simulink model "simscape_actuation_22_idealtorque"  (R2021a)
settings: Solver=VariableStepAuto  StartTime=0.001  StopTime=10  FixedStep=0.01  MaxStep=0.0001  RelTol=1e-4  AbsTol=1e-4
values from neighbouring files (symbols this model uses):
  As = 0.00025    [variables_5.mat]
  ext = 48232.2966308    [variables_5.mat]
  n = 0.912908754682    [variables_5.mat]
  ri = 0.00045    [variables_5.mat]
  ro = 0.0015    [variables_5.mat]
  Y = 7920.45919172    [variables_5.mat]
  yieldstress = 40000000    [variables_5.mat]
undefined symbols (not defined in the file or in its folder): Fac
libraries: fl_lib x18, sh_lib x11, nesl_utility x10, sdl_lib x2, pid_lib x1
settings Model: Creator=carme  LastModifiedBy=carme
settings SolverCC: AutoScaleAbsTol=off  AlgebraicLoopSolver=LineSearch
settings DebuggingCC: SymbolicDimsDataTypeCodeGenerationDiagnostic=none  SFMachineParentedDataDiag=warning
settings SFSimCC: CustomCodeUndefinedFunction=UseInterfaceOnly
settings SimscapeCC: SimscapeLogType=all  SimscapeLogSimulationStatistics=on  SimscapeLogDataHistory=10000

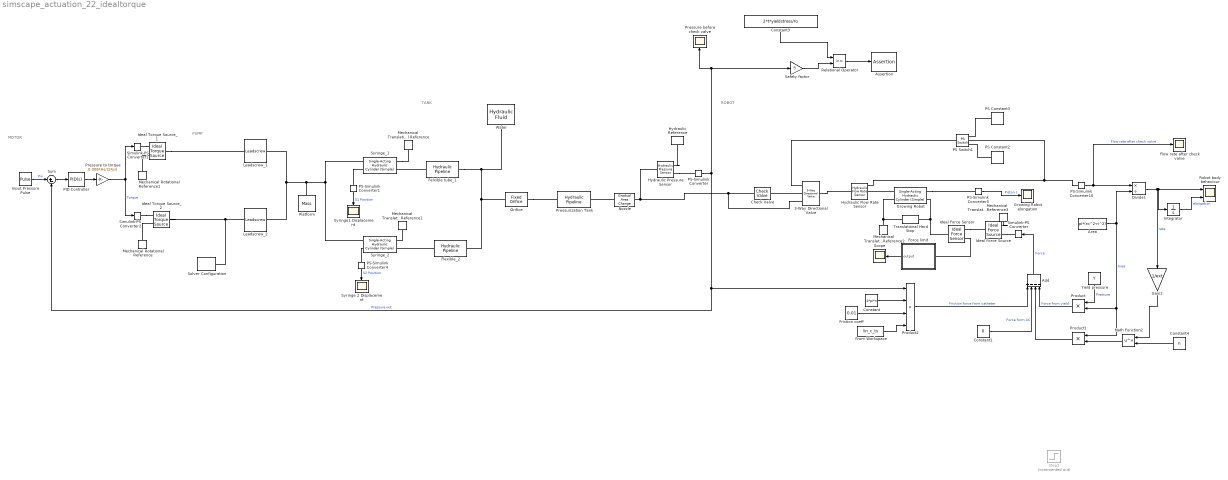
== system simscape_actuation_22_idealtorque ==
  note: MOTOR
  note: PUMP
  note: TANK
  note: ROBOT
  3-Way Directional Valve : sh_lib/Valves/Directional Valves/3-Way Directional Valve  area_spec=sh.valves.directional_valves.enum.area_spec.identical  x_0_P=0 m  x_0_T=0 m  mdl_type_identical=sh.valves.directional_valves.enum.mdl_type.linear  mdl_type_different=sh.valves.directional_valves.enum.mdl_type.linear  opening_max=0.005 m  area_max=0.5e-4 m^2  opening_max_P_A=0.005 m  area_max_P_A=0.5e-4 m^2  opening_max_A_T=0.005 m  area_max_A_T=0.5e-4 m^2  opening_area_tab=[-.002, 0, .002, .005, .015] m  area_tab=[1e-09, 2.0352e-07, 4.0736e-05, .00011438, .00034356] m^2  opening_flow_rate_tab=[-.002, 0, .002, .005, .015] m  pressure_tab=[-10000000, -5000000, -2000000, 2000000, 5000000, 10000000] Pa  flow_rate_tab=[-1e-07, -7.0711e-08, -4.4721e-08, 4.4721e-08, 7.0711e-08, 1e-07; -2.0352e-05, -1.4391e-05, -9.1017e-06, 9.1017e-06, 1.4391e-05, 2.0352e-05; -.0040736, -.0028805, -.0018218, .0018218, .0028805, .0040736; -.011438, -.0080879, -.0051152, .0051152, .0080879, .011438; -.034356, -.024293, -.015364, .015364, .024293, .034356] m^3/s  opening_area_tab_P_A=[-.002, 0, .002, .005, .015] m  area_tab_P_A=[1e-09, 2.0352e-07, 4.0736e-05, .00011438, .00034356] m^2  opening_flow_rate_tab_P_A=[-.002, 0, .002, .005, .015] m  pressure_tab_P_A=[-10000000, -5000000, -2000000, 2000000, 5000000, 10000000] Pa  flow_rate_tab_P_A=[-1e-07, -7.0711e-08, -4.4721e-08, 4.4721e-08, 7.0711e-08, 1e-07; -2.0352e-05, -1.4391e-05, -9.1017e-06, 9.1017e-06, 1.4391e-05, 2.0352e-05; -.0040736, -.0028805, -.0018218, .0018218, .0028805, .0040736; -.011438, -.0080879, -.0051152, .0051152, .0080879, .011438; -.034356, -.024293, -.015364, .015364, .024293, .034356] m^3/s  opening_area_tab_A_T=[-.002, 0, .002, .005, .015] m  area_tab_A_T=[1e-09, 2.0352e-07, 4.0736e-05, .00011438, .00034356] m^2  opening_flow_rate_tab_A_T=[-.002, 0, .002, .005, .015] m  pressure_tab_A_T=[-10000000, -5000000, -2000000, 2000000, 5000000, 10000000] Pa  flow_rate_tab_A_T=[-1e-07, -7.0711e-08, -4.4721e-08, 4.4721e-08, 7.0711e-08, 1e-07; -2.0352e-05, -1.4391e-05, -9.1017e-06, 9.1017e-06, 1.4391e-05, 2.0352e-05; -.0040736, -.0028805, -.0018218, .0018218, .0028805, .0040736; -.011438, -.0080879, -.0051152, .0051152, .0080879, .011438; -.034356, -.024293, -.015364, .015364, .024293, .034356] m^3/s  interp_method_identical=sh.valves.directional_valves.enum.interp_method.linear  interp_method_different=sh.valves.directional_valves.enum.interp_method.linear  extrap_method_identical=sh.valves.directional_valves.enum.extrap_method.linear  extrap_method_different=sh.valves.directional_valves.enum.extrap_method.linear  A_leak=1e-12 m^2  C_d=0.7  lam_spec=sh.valves.directional_valves.enum.lam_spec.pressure_ratio  B_lam=0.999  Re_cr=12
      settings: SourceProductBaseCode=SH  InternalSimscapePortConfiguration="{\"Bottom\":[],\"Left\":[{\"id\":\"A\",\"label\":\"A\",\"type\":\"foundation.hydraulic.hydraulic\"}],\"Right\":[{\"id\":\"S\",\"label\":\"S\",\"type\":\"input\"},{\"id\":\"P\",\"label\":\"P\",\"type\":\"foundation.hydraulic.hydraulic\"},{\"id\":\"T\",\"label\":\"T\",\"type\":\"foundation.hydraulic.hydraulic\"}],\"Top\":[]}"
  Add : Sum  Inputs=+---
  Area : Constant  Value=pi*(ro^2-ri^2)
  Assertion : Assertion  AssertionFailFcn=Yield failure
  Check Valve : sh_lib/Valves/Directional Valves/Check Valve  area_max=As m^2  pres_crack=Y Pa  pres_max=1.2e10 Pa  C_d=0.7  A_leak=1e-12 m^2  lam_spec=1  B_lam=0.999  Re_cr=12  dynamic=0  tau=0.1 s  area_init=1e-12 m^2
      settings: SourceProductBaseCode=SH  InternalSimscapePortConfiguration="{\"Bottom\":[],\"Left\":[{\"id\":\"A\",\"label\":\"A\",\"type\":\"foundation.hydraulic.hydraulic\"}],\"Right\":[{\"id\":\"B\",\"label\":\"B\",\"type\":\"foundation.hydraulic.hydraulic\"}],\"Top\":[]}"
  Constant : Constant  Value=2*pi*ri
  Constant1 : Constant  Value=0
  Constant3 : Constant  Value=2*t*yieldstress/ro
  Constant4 : Constant  Value=n
  Divide1 : Product  Inputs=*/
  Felxible tube_1 : sh_lib/Pipelines/Hydraulic Pipeline  cs_type=1  d_in=0.004 m  area=1e-4 m^2  D_h=1.12e-2 m  s_factor=64  length=0.3 m  length_ad=1 m  roughness=15e-6 m  Re_lam=2000  Re_turb=4000  wall_type=2  pr_r_coef=2e-12 m/Pa  time_const=0.01 s  k_sh=1.4  initial_pressure=200 Pa
      settings: SourceProductBaseCode=SH  InternalSimscapePortConfiguration="{\"Bottom\":[],\"Left\":[{\"id\":\"A\",\"label\":\"A\",\"type\":\"foundation.hydraulic.hydraulic\"}],\"Right\":[{\"id\":\"B\",\"label\":\"B\",\"type\":\"foundation.hydraulic.hydraulic\"}],\"Top\":[]}"
  Flexible_2 : sh_lib/Pipelines/Hydraulic Pipeline  cs_type=1  d_in=0.004 m  area=1e-4 m^2  D_h=1.12e-2 m  s_factor=64  length=0.3 m  length_ad=1 m  roughness=15e-6 m  Re_lam=2000  Re_turb=4000  wall_type=2  pr_r_coef=2e-12 m/Pa  time_const=0.01 s  k_sh=1.4  initial_pressure=200 Pa
      settings: SourceProductBaseCode=SH  InternalSimscapePortConfiguration="{\"Bottom\":[],\"Left\":[{\"id\":\"A\",\"label\":\"A\",\"type\":\"foundation.hydraulic.hydraulic\"}],\"Right\":[{\"id\":\"B\",\"label\":\"B\",\"type\":\"foundation.hydraulic.hydraulic\"}],\"Top\":[]}"
  Flow rate after check valve : Scope
  Force limit : Subsystem  mask{Flim=2}
      mask prompts: Flim "Force limit"
  Friction coeff : Constant  Value=0.01
  From Workspace : FromWorkspace  VariableName=lin_c_ts
  Gain2 : Gain  Gain=1/ext
  Growing Robot : sh_lib/Hydraulic Cylinders/Single-Acting Hydraulic Cylinder (Simple)  area=pi*(ro^2-ri^2) m^2  stroke=0.08 m  init_pos=0.01 m  penetr_coeff=1e12 s*N/m^2  or=1
      settings: SourceProductBaseCode=SH  InternalSimscapePortConfiguration="{\"Bottom\":[],\"Left\":[{\"id\":\"C\",\"label\":\"C\",\"type\":\"foundation.mechanical.translational.translational\"},{\"id\":\"A\",\"label\":\"A\",\"type\":\"foundation.hydraulic.hydraulic\"}],\"Right\":[{\"id\":\"R\",\"label\":\"R\",\"type\":\"foundation.mechanical.translational.translational\"},{\"id\":\"P\",\"label\":\"P\",\"type\":\"output\"}],\"Top\":[]}"
  Growing Robot elongation : Scope
  Hydraulic Flow Rate Sensor : fl_lib/Hydraulic/Hydraulic Sensors/Hydraulic Flow Rate Sensor
  Hydraulic Pressure Sensor : fl_lib/Hydraulic/Hydraulic Sensors/Hydraulic Pressure Sensor
  Hydraulic Reference : fl_lib/Hydraulic/Hydraulic Elements/Hydraulic Reference
  Ideal Force Sensor : fl_lib/Mechanical/Mechanical Sensors/Ideal Force Sensor
  Ideal Force Source : fl_lib/Mechanical/Mechanical Sources/Ideal Force Source
  Ideal Torque Source_1 : fl_lib/Mechanical/Mechanical Sources/Ideal Torque Source
  Ideal Torque Source_2 : fl_lib/Mechanical/Mechanical Sources/Ideal Torque Source
  Input Pressure Pulse : DiscretePulseGenerator  PulseType=Time based  Amplitude=150e3  Period=1.3  PulseWidth=90  PhaseDelay=0.26
  Integrator : Integrator
  Leadscrew_1 : sdl_lib/Gears/Rotational- Translational/Leadscrew  Lead=0.008 m  helix_type=sdl.enum.handedness.right  mu_visc=0.1 N*m/(rad/s)  friction_model=sdl.enum.gear_friction.none  friction_parameterization=sdl.enum.frictionParameterization.geometry  lambda=5 deg  alpha=17.5 deg  fr_coeff=0.05  eff_sn=0.75  eff_ns=0.45  temperature_TLU=[280, 300, 320] K  efficiency_sn_TLU=[.75, .65, .6]  efficiency_ns_TLU=[.5, .45, .4]  pwr_thr=0.001 W  thermal_mass=50 J/K  temperature_specify=off  temperature_priority=High  temperature=300 K  temperature_nominal_specify=off  temperature_nominal_unit=K  temperature_nominal_value=1
      settings: SourceProductBaseCode=LD  InternalSimscapePortConfiguration="{\"Bottom\":[],\"Left\":[{\"id\":\"S\",\"label\":\"S\",\"type\":\"foundation.mechanical.rotational.rotational\"}],\"Right\":[{\"id\":\"N\",\"label\":\"N\",\"type\":\"foundation.mechanical.translational.translational\"}],\"Top\":[]}"
  Leadscrew_2 : sdl_lib/Gears/Rotational- Translational/Leadscrew  Lead=0.008 m  helix_type=sdl.enum.handedness.right  mu_visc=0.1 N*m/(rad/s)  friction_model=sdl.enum.gear_friction.none  friction_parameterization=sdl.enum.frictionParameterization.geometry  lambda=5 deg  alpha=17.5 deg  fr_coeff=0.05  eff_sn=0.75  eff_ns=0.45  temperature_TLU=[280, 300, 320] K  efficiency_sn_TLU=[.75, .65, .6]  efficiency_ns_TLU=[.5, .45, .4]  pwr_thr=0.001 W  thermal_mass=50 J/K  temperature_specify=off  temperature_priority=High  temperature=300 K  temperature_nominal_specify=off  temperature_nominal_unit=K  temperature_nominal_value=1
      settings: SourceProductBaseCode=LD  InternalSimscapePortConfiguration="{\"Bottom\":[],\"Left\":[{\"id\":\"S\",\"label\":\"S\",\"type\":\"foundation.mechanical.rotational.rotational\"}],\"Right\":[{\"id\":\"N\",\"label\":\"N\",\"type\":\"foundation.mechanical.translational.translational\"}],\"Top\":[]}"
  Math Function2 : Math  Operator=pow  SignedPower=on  SaturateOnIntegerOverflow=on
  Mechanical Rotational Reference : fl_lib/Mechanical/Rotational Elements/Mechanical Rotational Reference
  Mechanical Rotational Reference1 : fl_lib/Mechanical/Rotational Elements/Mechanical Rotational Reference
  Mechanical Translational Reference{,1..3} (4 alike) : fl_lib/Mechanical/Translational Elements/Mechanical Translational Reference
  Nozzle : sh_lib/Local Hydraulic Resistances/Gradual Area Change  mdl_type=1  small_diam=0.002 m  large_diam=0.015 m  angle=30 deg  kp_c=1  lam_spec=1  B_lam=0.999  Re_cr=350  Re_vec=[-10000, -5000, -4000, -2000, -1000, -500, -200, -100, -50, -40, -30, -20, -10, 10, 20, 30, 40, 50, 100, 200, 500, 1000, 2000, 4000, 5000, 10000]  loss_coeff_vec=[.05, .05, .06, .09, .15, .26, .4, .61, .91, 1.12, 1.48, 2.23, 4.4, 4, 1.9, 1.26, .94, .76, .52, .48, .42, .36, .24, .4, .42, .35]  interp_method=1  extrap_method=1
      settings: SourceProductBaseCode=SH  InternalSimscapePortConfiguration="{\"Bottom\":[],\"Left\":[{\"id\":\"A\",\"label\":\"A\",\"type\":\"foundation.hydraulic.hydraulic\"}],\"Right\":[{\"id\":\"B\",\"label\":\"B\",\"type\":\"foundation.hydraulic.hydraulic\"}],\"Top\":[]}"
  Orifice : sh_lib/Orifices/Fixed Orifice  area=1.2566e-5 m^2  C_d=0.7  lam_spec=1  B_lam=0.999  Re_cr=12  q_specify=off  q_priority=None  q=0.001 m^3/s  q_nominal_specify=off  q_nominal_unit=m^3/s  q_nominal_value=1  p_specify=off  p_priority=None  p=0 Pa  p_nominal_specify=off  p_nominal_unit=Pa  p_nominal_value=1
      settings: SourceProductBaseCode=SH  InternalSimscapePortConfiguration="{\"Bottom\":[],\"Left\":[{\"id\":\"A\",\"label\":\"A\",\"type\":\"foundation.hydraulic.hydraulic\"}],\"Right\":[{\"id\":\"B\",\"label\":\"B\",\"type\":\"foundation.hydraulic.hydraulic\"}],\"Top\":[]}"
  PID Controller : pid_lib/PID Controller  Controller=PID  Form=Parallel  TimeDomain=Continuous-time  UseExternalTs=off  SampleTime=-1  IntegratorMethod=Forward Euler  FilterMethod=Forward Euler  ControllerParametersSource=internal  P=20  I=80  D=0.5  UseFilter=on  N=100  TunerSelectOption=Transfer Function Based (PID Tuner App)  InitialConditionSource=internal  InitialConditionForIntegrator=0  InitialConditionForFilter=0  DifferentiatorICPrevScaledInput=0  ExternalReset=none  TrackingMode=off  Kt=1  LimitOutput=off  SatLimitsSource=internal  UpperSaturationLimit=inf  LowerSaturationLimit=-inf  LinearizeAsGain=on  AntiWindupMode=none  Kb=1  POutMin=[]  POutMax=[]  IOutMin=[]  IOutMax=[]  DOutMin=[]  DOutMax=[]  NOutMin=[]  NOutMax=[]  SumOutMin=[]  SumOutMax=[]  SaturationOutMin=[]  SaturationOutMax=[]  PParamMin=[]  PParamMax=[]  IParamMin=[]  IParamMax=[]  DParamMin=[]  DParamMax=[]  NParamMin=[]  NParamMax=[]  KbParamMin=[]  KbParamMax=[]  KtParamMin=[]  KtParamMax=[]  KbOutMin=[]  KbOutMax=[]  KtOutMin=[]  KtOutMax=[]  IntegratorOutMin=[]  IntegratorOutMax=[]  FilterOutMin=[]  FilterOutMax=[]  SumI1OutMin=[]  SumI1OutMax=[]  SumI2OutMin=[]  SumI2OutMax=[]  SumI3OutMin=[]  SumI3OutMax=[]  SumI4OutMin=[]  SumI4OutMax=[]  SumDOutMin=[]  SumDOutMax=[]  DifferentiatorOutMin=[]  DifferentiatorOutMax=[]  FilterDiffOutCoefMin=[]  FilterDiffOutCoefMax=[]  ReciprocalOutMin=[]  ReciprocalOutMax=[]  SumDenOutMin=[]  SumDenOutMax=[]  SumNumOutMin=[]  SumNumOutMax=[]  DivideOutMin=[]  DivideOutMax=[]  UdiffTsProdOutMin=[]  UdiffTsProdOutMax=[]  NTsProdOutMin=[]  NTsProdOutMax=[]  UintegralTsProdOutMin=[]  UintegralTsProdOutMax=[]  UngainTsProdOutMin=[]  UngainTsProdOutMax=[]  IntegratorContinuousStateAttributes=''  IntegratorStateMustResolveToSignalObject=off  IntegratorRTWStateStorageClass=Auto  FilterContinuousStateAttributes=''  FilterStateMustResolveToSignalObject=off  FilterRTWStateStorageClass=Auto  ParallelPVariant=InternalParameters  IdealPVariant=Disabled  IVariant=InternalParameters  DVariant=InternalParameters  IntegratorVariant=Continuous  SatVariant=Disabled  AWVariant=Passthrough  PCopyVariant=Disabled  TRVariant=Disabled  FdbkBlocksVariant=Forward  IdealPFdbkVariant=Disabled  SatFdbkVariant=Disabled  DerivativeFilterVariant=ContFilter  NVariant=InternalParameters  NCopyVariant=Disabled  FilterICVariant=InternalICsFilter  IntegratorICVariant=InternalICs  ExternalResetVariant=Disabled  TRSumVariant=Passthrough  SumFdbkVariant=Disabled  SumVariant=Sum_PID  TsampFilterVariant=InternalTs  TsampNgainVariant=Passthrough  TsampIntegralVariant=Passthrough  ExternalSaturationOutDataTypeStr=Inherit: Same as second input
  PS Constant2 : fl_lib/Physical Signals/Sources/PS Constant  constant=1
  PS Constant3 : fl_lib/Physical Signals/Sources/PS Constant  constant=-1
  PS Switch1 : fl_lib/Physical Signals/Nonlinear Operators/PS Switch  Threshold=0 m^3/s
      settings: SourceProductBaseCode=SS  InternalSimscapePortConfiguration="{\"Bottom\":[],\"Left\":[{\"id\":\"I1\",\"label\":\"\",\"type\":\"input\"},{\"id\":\"I2\",\"label\":\"\",\"type\":\"input\"},{\"id\":\"I3\",\"label\":\"\",\"type\":\"input\"}],\"Right\":[{\"id\":\"O\",\"label\":\"\",\"type\":\"output\"}],\"Top\":[]}"
  PS-Simulink Converter{,1,4..5,10} (5 alike) : nesl_utility/PS-Simulink Converter  PhysicalDomain=network_engine_domain  SubClassName=ps_output  LeftPortType=input  RightPortType=output  PseudoPeriodic=off  Frequencies=[]  Unit=inherit  AffineConversion=off
      PS-Simulink Converter settings: SourceProductName=Utilities
      PS-Simulink Converter1 settings: SourceProductName=Utilities
      PS-Simulink Converter10 settings: SourceProductName=Utilities
      PS-Simulink Converter4 settings: SourceProductName=Utilities
      PS-Simulink Converter5 settings: SourceProductBaseCode=PW,SS
  Platform : fl_lib/Mechanical/Translational Elements/Mass  mass=0.001 kg  num_ports=foundation.enum.numPorts2.one  v_specify=off  v_priority=High  v=0 m/s  v_nominal_specify=off  v_nominal_unit=m/s  v_nominal_value=1  f_specify=off  f_priority=None  f=0 N  f_nominal_specify=off  f_nominal_unit=N  f_nominal_value=1
  Pressure before check valve : Scope
  Pressure to torque : Gain  Gain=0.008*As/(2*pi)
  Pressurization Tank : sh_lib/Pipelines/Hydraulic Pipeline  cs_type=2  d_in=0.25 m  area=1.695e-4 m^2  D_h=15e-3 m  s_factor=64  length=0.122 m  length_ad=1 m  roughness=15e-6 m  Re_lam=2000  Re_turb=4000  wall_type=1  pr_r_coef=2e-12 m/Pa  time_const=0.01 s  k_sh=1.4  initial_pressure=1 Pa
      settings: SourceProductBaseCode=SH  InternalSimscapePortConfiguration="{\"Bottom\":[],\"Left\":[{\"id\":\"A\",\"label\":\"A\",\"type\":\"foundation.hydraulic.hydraulic\"}],\"Right\":[{\"id\":\"B\",\"label\":\"B\",\"type\":\"foundation.hydraulic.hydraulic\"}],\"Top\":[]}"
  Product : Product
  Product1 : Product
  Product2 : Product  Inputs=4
  Relational Operator : RelationalOperator  OutDataTypeStr=boolean  RndMeth=Simplest
  Robot body behaviour : Scope  NumInputPorts=2
  Safety factor : Gain  Gain=5
  Scope : Scope
  Simulink-PS Converter : nesl_utility/Simulink-PS Converter  PhysicalDomain=network_engine_domain  SubClassName=ps_input  LeftPortType=input  RightPortType=output  PseudoPeriodic=off  Frequencies=[]  NoiseDistribution=none  NoiseParameters=[]  Unit=1  AffineConversion=off  FilteringAndDerivatives=provide  SimscapeFilterOrder=1  InputFilterTimeConstant=0.001  UdotUserProvided=0
      settings: SourceProductBaseCode=PW,SS
  Simulink-PS Converter1 : nesl_utility/Simulink-PS Converter  PhysicalDomain=network_engine_domain  SubClassName=ps_input  LeftPortType=input  RightPortType=output  PseudoPeriodic=off  Frequencies=[]  NoiseDistribution=none  NoiseParameters=[]  Unit=1  AffineConversion=off  FilteringAndDerivatives=provide  SimscapeFilterOrder=1  InputFilterTimeConstant=0.001  UdotUserProvided=0
      settings: SourceProductBaseCode=PW,SS
  Simulink-PS Converter2 : nesl_utility/Simulink-PS Converter  PhysicalDomain=network_engine_domain  SubClassName=ps_input  LeftPortType=input  RightPortType=output  PseudoPeriodic=off  Frequencies=[]  NoiseDistribution=none  NoiseParameters=[]  Unit=1  AffineConversion=off  FilteringAndDerivatives=provide  SimscapeFilterOrder=1  InputFilterTimeConstant=0.001  UdotUserProvided=0
      settings: SourceProductBaseCode=PW,SS
  Solver Configuration : nesl_utility/Solver Configuration  PhysicalDomain=network_engine_domain  SubClassName=solver  LeftPortType=input  RightPortType=generic  Tones=[]  Harmonics=[]  SimulateNoise=off  Profile=off  UseLocalSampling=off  EnableSwitchedLinearOptims=on  FrequencyDomain=off  UseCCode=off  RelTol=0.001  AbsTol=1e-06  MinStep=1e-09  ToWorkspace=off  RevertToSquareIcSolve=off  NumHomotopyIterations=100  PhasorMode=off  PhasorModeNumHarmonics=1  DoDC=off  ResidualTolerance=1e-09  UseLocalSolver=off  LocalSolverChoice=NE_BACKWARD_EULER_ADVANCER  LocalSolverSampleTime=0.001  DoFixedCost=off  MaxNonlinIter=3  MaxModeIter=2  ComputeImpulses=off  ImpulseIterations=2  LinearAlgebra=auto  EquationFormulation=NE_TIME_EF  DelaysMemoryBudget=1024  AutomaticFiltering=on  FilteringTimeConstant=0.001  PartitionStorageMethod=AS_NEEDED  PartitionMemoryBudget=1024  PartitionMethod=ROBUST
      settings: SourceProductBaseCode=PW,SS
  Step1 : Step  Commented=on  After=Fac  SampleTime=0
  Sum : Sum  Inputs=|+-
  Syringe 2 Displacement : Scope
  Syringe1 Displacement : Scope
  Syringe_1 : sh_lib/Hydraulic Cylinders/Single-Acting Hydraulic Cylinder (Simple)  area=As m^2  stroke=0.05 m  init_pos=0.05 m  penetr_coeff=1e12 s*N/m^2  or=2
      settings: SourceProductBaseCode=SH  InternalSimscapePortConfiguration="{\"Bottom\":[],\"Left\":[{\"id\":\"C\",\"label\":\"C\",\"type\":\"foundation.mechanical.translational.translational\"},{\"id\":\"A\",\"label\":\"A\",\"type\":\"foundation.hydraulic.hydraulic\"}],\"Right\":[{\"id\":\"R\",\"label\":\"R\",\"type\":\"foundation.mechanical.translational.translational\"},{\"id\":\"P\",\"label\":\"P\",\"type\":\"output\"}],\"Top\":[]}"
  Syringe_2 : sh_lib/Hydraulic Cylinders/Single-Acting Hydraulic Cylinder (Simple)  area=As m^2  stroke=0.05 m  init_pos=0.05 m  penetr_coeff=1e12 s*N/m^2  or=2
      settings: SourceProductBaseCode=SH  LogSimulationData=on  InternalSimscapePortConfiguration="{\"Bottom\":[],\"Left\":[{\"id\":\"C\",\"label\":\"C\",\"type\":\"foundation.mechanical.translational.translational\"},{\"id\":\"A\",\"label\":\"A\",\"type\":\"foundation.hydraulic.hydraulic\"}],\"Right\":[{\"id\":\"R\",\"label\":\"R\",\"type\":\"foundation.mechanical.translational.translational\"},{\"id\":\"P\",\"label\":\"P\",\"type\":\"output\"}],\"Top\":[]}"
  "Translational Hard Stop " : fl_lib/Mechanical/Translational Elements/Translational Hard Stop  upper_bnd=0.08 m  lower_bnd=-0.08 m  stiff_up=1e6 N/m  stiff_low=1e6 N/m  D_up=150 N/(m/s)  D_low=150 N/(m/s)  model=simscape.enum.hardstop.smooth  transition=0.1 mm  v_specify=off  v_priority=None  v=0 m/s  v_nominal_specify=off  v_nominal_unit=m/s  v_nominal_value=1  f_specify=off  f_priority=None  f=0 N  f_nominal_specify=off  f_nominal_unit=N  f_nominal_value=1  x_specify=off  x_priority=High  x=0 m  x_nominal_specify=off  x_nominal_unit=m  x_nominal_value=1
  Water : sh_lib/Hydraulic Utilities/Hydraulic Fluid  DataSource=1  SelFluid=24  SysTemp=22  TrapAir=0.005  ViscDerFactor=1  range_error=2
  Yield pressure : Constant  Value=Y
  wires:
  PS-Simulink Converter1/1 -> Syringe1 Displacement/1  "S1 Position"
  PS-Simulink Converter4/1 -> Syringe 2 Displacement/1  "S2 Position"
  PS-Simulink Converter/1 -> Safety factor/1, Pressure before check valve/1, Product2/1, Sum/2  "Pressure out"
  Integrator/1 -> Robot body behaviour/2  "elongation"
  PS-Simulink Converter10/1 -> Flow rate after check valve/1, Divide1/1  "Flow rate after check valve"
  Add/1 -> Simulink-PS Converter/1  "Force"
  Yield pressure/1 -> Product/1  "Pressure"
  Product/1 -> Add/4  "Force from yield"
  Constant1/1 -> Add/2  "Force form AC"
  Constant/1 -> Product2/2
  Friction coeff/1 -> Product2/3
  Product2/1 -> Add/1  "Friction force from catheter"
  Input Pressure Pulse/1 -> Sum/1  "Pin"
  Pressure to torque/1 -> Simulink-PS Converter2/1, Simulink-PS Converter1/1  "Torque"
  Sum/1 -> PID Controller/1
  PID Controller/1 -> Pressure to torque/1
  PS-Simulink Converter5/1 -> Growing Robot elongation/1  "Piston L"
  From Workspace/1 -> Product2/4
  Relational Operator/1 -> Assertion/1
  Constant3/1 -> Relational Operator/1
  Area/1 -> Product1/1, Product/2, Divide1/2  "Area"
  Divide1/1 -> Robot body behaviour/1, Integrator/1, Gain2/1  "rate"
  Gain2/1 -> Math Function2/1
  Product1/1 -> Add/3
  Math Function2/1 -> Product1/2
  Constant4/1 -> Math Function2/2
  Force limit/1(output) -> Scope/1
  Safety factor/1 -> Relational Operator/2
  connections:
  PS-Simulink Converter1/LConn1 -- Syringe_1/RConn2
  Syringe_1/LConn1 -- Mechanical Translational Reference/LConn1
  Syringe_2/LConn1 -- Mechanical Translational Reference1/LConn1
  PS-Simulink Converter4/LConn1 -- Syringe_2/RConn2
  Leadscrew_1/RConn1 -- Leadscrew_2/RConn1 -- Syringe_2/RConn1 -- Syringe_1/RConn1 -- Platform/LConn1
  Nozzle/RConn1 -- Pressurization Tank/RConn1
  Felxible tube_1/LConn1 -- Syringe_1/LConn2
  Ideal Torque Source_1/LConn1 -- Leadscrew_1/LConn1
  Hydraulic Pressure Sensor/RConn2 -- PS-Simulink Converter/LConn1
  Hydraulic Pressure Sensor/RConn1 -- Hydraulic Reference/LConn1
  Orifice/RConn1 -- Pressurization Tank/LConn1
  Felxible tube_1/RConn1 -- Water/RConn1 -- Flexible_2/RConn1 -- Orifice/LConn1
  Flexible_2/LConn1 -- Syringe_2/LConn2
  Ideal Torque Source_2/LConn1 -- Solver Configuration/RConn1 -- Leadscrew_2/LConn1
  Ideal Torque Source_2/RConn2 -- Mechanical Rotational Reference/LConn1
  Ideal Torque Source_1/RConn2 -- Mechanical Rotational Reference1/LConn1
  Hydraulic Flow Rate Sensor/RConn1 -- PS-Simulink Converter10/LConn1 -- PS Switch1/LConn2
  Growing Robot/LConn2 -- Hydraulic Flow Rate Sensor/RConn2
  Mechanical Translational Reference2/LConn1 -- Growing Robot/LConn1 -- "Translational Hard Stop "/RConn1
  Ideal Force Source/RConn2 -- Mechanical Translational Reference3/LConn1
  Ideal Force Source/RConn1 -- Simulink-PS Converter/RConn1
  Growing Robot/RConn2 -- PS-Simulink Converter5/LConn1
  Simulink-PS Converter2/RConn1 -- Ideal Torque Source_2/RConn1
  Simulink-PS Converter1/RConn1 -- Ideal Torque Source_1/RConn1
  "Translational Hard Stop "/LConn1 -- Growing Robot/RConn1 -- Ideal Force Sensor/LConn1
  3-Way Directional Valve/LConn1 -- Hydraulic Flow Rate Sensor/LConn1
  PS Switch1/RConn1 -- 3-Way Directional Valve/RConn1
  Nozzle/LConn1 -- Check Valve/LConn1 -- 3-Way Directional Valve/RConn3 -- Hydraulic Pressure Sensor/LConn1
  3-Way Directional Valve/RConn2 -- Check Valve/RConn1
  PS Constant3/RConn1 -- PS Switch1/LConn3
  PS Constant2/RConn1 -- PS Switch1/LConn1
  Ideal Force Sensor/RConn1 -- Ideal Force Source/LConn1
  Ideal Force Sensor/RConn2 -- Force limit/LConn1

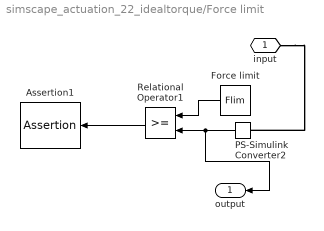
== system simscape_actuation_22_idealtorque/Force limit ==
  Assertion1 : Assertion  AssertionFailFcn=Force limit exceeded  StopWhenAssertionFail=off
  Force limit : Constant  Value=Flim
  PS-Simulink Converter2 : nesl_utility/PS-Simulink Converter  PhysicalDomain=network_engine_domain  SubClassName=ps_output  LeftPortType=input  RightPortType=output  PseudoPeriodic=off  Frequencies=[]  Unit=inherit  AffineConversion=off
      settings: SourceProductBaseCode=PW,SS
  Relational Operator1 : RelationalOperator  OutDataTypeStr=boolean  RndMeth=Simplest
  input : PMIOPort  Side=Left
  output : Outport
  wires:
  PS-Simulink Converter2/1 -> output/1, Relational Operator1/2
  Relational Operator1/1 -> Assertion1/1
  Force limit/1 -> Relational Operator1/1
  connections:
  input/RConn1 -- PS-Simulink Converter2/LConn1
